simulink subsystem "PvtSubSys_VIE"  (R2020b)
settings: Solver=VariableStepAuto  StartTime=0.0  StopTime=10.0  RelTol=1e-3
undefined symbols (not defined in the file): P_Global_CharSpd_ms, P_Global_FrontAxleToCenter_m, P_Global_RearAxleToCenter_m, P_Global_SideSlipAnglefactor, P_Global_SteeringAngleRatio, P_Global_WheelBase_m, P_Global_WheelTrack_m
libraries: simulink x16
(part 2 of 2)

== matlab function PvtSubSys_VIE/VIE/VIE/VxvRef_Calc/transBrakeToDrive ==
  data: l_tTransBrakeToDrive output; l_tTransDriveToBrake output; axvRefK1 input; axvRef input; vxvRef input; l_tTransBrakeToDriveK1 input single; l_tTransDriveToBrakeK1 input single; l_tHysARefDriveToBrakeInput input single; l_tHysARefBrakeToDriveInput input single; l_tHysARefDriveToBrakeOutput output; l_tHysARefBrakeToDriveOutput output
function [l_tTransBrakeToDrive,l_tTransDriveToBrake,l_tHysARefDriveToBrakeOutput,l_tHysARefBrakeToDriveOutput] = fcn(axvRefK1,axvRef,vxvRef,l_tTransBrakeToDriveK1,l_tTransDriveToBrakeK1,l_tHysARefDriveToBrakeInput,l_tHysARefBrakeToDriveInput)
%#codegen
l_tTransBrakeToDrive = max((l_tTransBrakeToDriveK1-single(0.02)),single(0));  % 常数值转为single型
l_tTransDriveToBrake = max((l_tTransDriveToBrakeK1-single(0.02)),single(0));  % 常数值转为single型

l_tHysARefDriveToBrake=l_tHysARefDriveToBrakeInput;
l_tHysARefBrakeToDrive=l_tHysARefBrakeToDriveInput;

% vsp_checkReinitHys_V
if ((axvRefK1>-0.3)&&(axvRef>-0.3)&&(vxvRef>0))||((axvRefK1<0.3)&&(axvRef<0.3)&&(vxvRef<0)) 
    l_tHysARefDriveToBrake=single(0);% 常数值转为single型
    l_tHysARefBrakeToDrive=single(0);% 常数值转为single型
end
if ((axvRefK1<-0.7)&&(axvRef<-0.7)&&(vxvRef>0))||((axvRefK1>0.7)&&(axvRef>0.7)&&(vxvRef<0)) 
    l_tHysARefDriveToBrake=single(0);% 常数值转为single型
    l_tHysARefBrakeToDrive=single(0);% 常数值转为single型
end   

% vsp_checkStartHys_V
if ((axvRefK1>=-0.3)&&(axvRef<-0.3)&&(vxvRef>0))||((axvRefK1<=0.3)&&(axvRef>0.3)&&(vxvRef<0)) 
   l_tHysARefDriveToBrake = l_tHysARefDriveToBrake + single(0.02);% 常数值转为single型
end
if ((axvRefK1<=-0.7)&&(axvRef>-0.7)&&(vxvRef>0))||((axvRefK1>=0.7)&&(axvRef<0.7)&&(vxvRef<0)) 
   l_tHysARefBrakeToDrive = l_tHysARefBrakeToDrive + single(0.02);% 常数值转为single型
end  

% vsp_checkIncrHys_V
if ((axvRef>=-0.7)&&(axvRef<=-0.3)&&(vxvRef>0))||((axvRef<=0.7)&&(axvRef>=0.3)&&(vxvRef<0)) 
    if l_tHysARefDriveToBrake>0
        l_tHysARefDriveToBrake = min((l_tHysARefDriveToBrake + single(0.02)),single(0.16));% 常数值转为single型
    end
    if l_tHysARefBrakeToDrive>0
        l_tHysARefBrakeToDrive = min((l_tHysARefBrakeToDrive + single(0.02)),single(0.16));% 常数值转为single型
    end
end
%-----------------------------------------------------------------------------------------------%
if ((axvRefK1>=-0.7)&&(axvRef<-0.7)&&(vxvRef>0))||((axvRefK1<=0.7)&&(axvRef>0.7)&&(vxvRef<0))
    if (l_tHysARefDriveToBrake>0)&&(l_tHysARefDriveToBrake<0.16)
        l_tTransDriveToBrake = single(0.15);% 常数值转为single型
    end
end
if ((axvRefK1<=-0.3)&&(axvRef>-0.3)&&(vxvRef>0))||((axvRefK1>=0.3)&&(axvRef<0.3)&&(vxvRef<0))
    if (l_tHysARefBrakeToDrive>0)&&(l_tHysARefBrakeToDrive<0.16)
        l_tTransBrakeToDrive = single(0.15);% 常数值转为single型
    end
end

    l_tHysARefDriveToBrakeOutput=l_tHysARefDriveToBrake;
    l_tHysARefBrakeToDriveOutput=l_tHysARefBrakeToDrive;

== matlab function PvtSubSys_VIE/VIE/VIE/VxvRef_Calc/vsp_calcNoCali_v ==
  data: vxvRef output single; vxwMeanIn input single; l_vxvRefMean input; axvRefLP input single; VehicleStandstill input; axvRefK1 input; axvRef output single
function [vxvRef,axvRef]   = fcn(vxwMeanIn,l_vxvRefMean,axvRefLP,VehicleStandstill,axvRefK1)
%#codegen
vxvRef = l_vxvRefMean;
t_AbsVxwMeanIn = abs(vxwMeanIn);

if t_AbsVxwMeanIn <=0.0039   %%%
    if VehicleStandstill==uint8(1)%转换常数数据类型
        vxvRef=single(0);%转换常数数据类型
        axvRef=single(0);%转换常数数据类型
    else
        axvRef = axvRefK1-single(0.1)*axvRefK1;%转换常数数据类型
    end
else
    axvRef = axvRefLP;
end

== matlab function PvtSubSys_VIE/VIE/VIE/VxvRef_Calc/vsp_filtVxvRefRaw ==
  data: Init input uint8; t_vxvRefRaw input; l_vxvRef input; l_CaseDrive input; l_CaseBrake input; l_tTransDriveToBrake input; l_tTransBrakeToDrive input; vxvRefRaw output; vxvRefRawK1 input single
function vxvRefRaw   = fcn(Init,t_vxvRefRaw,l_vxvRef,l_CaseDrive,l_CaseBrake,l_tTransDriveToBrake,l_tTransBrakeToDrive,vxvRefRawK1)
%#codegen
tFilter=single(1);%转换常数数据类型

if Init==uint8(0)%转换常数数据类型
    if (l_CaseDrive==uint8(0))&&(l_CaseBrake==uint8(0))%转换常数数据类型
        tFilter=single(0.25);%转换常数数据类型
    end
    if (l_tTransDriveToBrake>0)||(l_tTransBrakeToDrive>0)%转换常数数据类型
        tFilter=single(0.125);%转换常数数据类型
    end

    vxvRefRaw = vxvRefRawK1 + tFilter*(t_vxvRefRaw - vxvRefRawK1);

    t_temp1 = abs(vxvRefRaw);
    t_temp2 = abs(l_vxvRef);

    if ((l_CaseBrake==uint8(1))&&(t_temp1>t_temp2))||((l_CaseDrive==uint8(1))&&(t_temp1<t_temp2))%转换常数数据类型
       vxvRefRaw = l_vxvRef;
    end


    t_temp1 = single(0.24);%转换常数数据类型
    t_temp2 = vxvRefRawK1 + t_temp1;
    t_temp3 = vxvRefRawK1 - t_temp1;

    t_temp1 = min(vxvRefRaw,t_temp2);
    vxvRefRaw = max(t_temp1,t_temp3);
else
    vxvRefRaw = t_vxvRefRaw;
end

== matlab function PvtSubSys_VIE/VIE/VIE/alpSumSlideCurveness ==
  data: vRef input; alpSumSlideCurveness output; psiDtOpt input; alpSumSlideCurvenessK1 input single
function alpSumSlideCurveness = fcn(vRef,psiDtOpt,alpSumSlideCurvenessK1)

if abs(vRef)<0.01
   t_tauCurveness = single(65535);%转换常数数据类型
else
   t_tauCurveness = min(400/abs(vRef),single(65535));%转换常数数据类型
end
% t_tauKapDtCurvenessUp = t_tauCurveness/8;
% t_tauKapDtCurvenessDown = t_tauCurveness/2;

temp1 = single(abs(psiDtOpt));%abs(psiDtOpt)转为single型
if temp1<0.003
   temp1 = single(0); %转换常数数据类型
end
temp2 = alpSumSlideCurvenessK1/t_tauCurveness;
temp2 = temp1 - temp2;
temp3 = single(0.02)*temp2;%转换常数数据类型
alpSumSlideCurveness = min(alpSumSlideCurvenessK1 + temp3,single(2));%转换常数数据类型

end

== matlab function PvtSubSys_VIE/VIE/VIE/VxvRef_Calc/VxvRef_Calc/MATLAB Function2 ==
  data: y output; SteerAngleOffset_deg input single; SteerAngOffsetInit input single
function y  = fcn(SteerAngleOffset_deg,SteerAngOffsetInit)

persistent T
if isempty(T)
    T = single(0);
end

t = single(0.02);
T = min(T+t,1000);
if T > 0.1
    y = SteerAngleOffset_deg;       
else
    y = SteerAngOffsetInit;
end

end

== matlab function PvtSubSys_VIE/VIE/VIE/AxRef/MATLAB Function ==
  data: AxvS input; Ax output; AxvRef input; VxvRef input; Error input; AxK1 input single
function Ax = fcn(AxvS,AxvRef,VxvRef,Error,AxK1)
%#codegen
if (AxvRef==uint8(0))&&(VxvRef==uint8(0))%转换常数数据类型
    Ax=single(0);%转换常数数据类型
else
   if abs(AxvS-AxvRef)<Error
       AxRaw = single(0.5)*(AxvS+AxvRef);%转换常数数据类型
   else
       AxRaw = AxvRef;
   end
    Ax = single(0.25)*(AxRaw-AxK1) + AxK1;%转换常数数据类型
end

== matlab function PvtSubSys_VIE/VIE/VIE/PsiDtStandstillCalc/MATLAB Function ==
  data: AlpDtSteerAngle input single; PsiDtLP output single; PsiDtInF input single; Standstill input boolean; PsiDtDt input; PsiDtDtLP input single; PsiDtLPK1 input; PsiDtStandstillK1 input; PsiDtStandstill output single
function [PsiDtLP,PsiDtStandstill] = PsiDtStandstillCalc(AlpDtSteerAngle,PsiDtInF,Standstill,PsiDtDt,PsiDtDtLP,PsiDtLPK1,PsiDtStandstillK1)
%#codegen
PsiDtStandstill = PsiDtStandstillK1;
PsiDtLP = PsiDtLPK1;
tauLPStill = single(0.02)/single(0.5);%转换常数数据类型
tauLPStandStill = single(0.02)/single(5);%转换常数数据类型
PsiDtLP = PsiDtLP + tauLPStill*(PsiDtInF-PsiDtLP);
if (Standstill==1)&&...
        (abs(PsiDtLP)<0.08)&&...
        (abs(PsiDtDt)<0.1)&&...
        (abs(PsiDtDtLP)<0.01)&&...
        (abs(AlpDtSteerAngle)<=1.5708)
    PsiDtStandstill = PsiDtStandstill + tauLPStandStill*(PsiDtInF-PsiDtStandstill);
end

== matlab function PvtSubSys_VIE/VIE/VIE/VxvRef_Calc/VxvRef_Calc/YOD_Ackman ==
  data: AckConst output; VxvRef input; Vch input; WheelBase input; AlpWheelAngle input; PsiDtAckK1 input single; PsiDtAck output
function [AckConst,PsiDtAck] = Ackman(VxvRef,Vch,WheelBase,AlpWheelAngle,PsiDtAckK1)
%#codegen
if VxvRef==uint8(0)%转换常数数据类型
    PsiDtAckRaw = single(0);%转换常数数据类型
    AckConst = single(1);%转换常数数据类型
else
    AckConst = min((single(1)+VxvRef*VxvRef/(Vch*Vch))*WheelBase/VxvRef,single(32767));%转换常数数据类型
    PsiDtAckRaw = AlpWheelAngle/AckConst;
end
PsiDtAck = (single(0.02/0.1))*(PsiDtAckRaw-PsiDtAckK1)+PsiDtAckK1;%转换常数数据类型

== matlab function PvtSubSys_VIE/VIE/VIE/VxvRef_Calc/VxwCorr ==
  data: VxwFL input single; vxwCorrFL output; VxwFR input single; VxwRL input single; VxwRR input single; L1 input; L2 input; Yawrate input; alpAngle input; b input; vxwCorrFR output; vxwCorrRL output; vxwCorrRR output
function [vxwCorrFL,vxwCorrFR,vxwCorrRL,vxwCorrRR] = fcn(VxwFL,VxwFR,VxwRL,VxwRR,L1,L2,Yawrate,alpAngle,b)
%#codegen

vxwCorrFL = (VxwFL-(L1+L2)*Yawrate*sin(alpAngle))/cos(alpAngle) + b*Yawrate/single(2); %常数转为single类型

vxwCorrFR = (VxwFR-(L1+L2)*Yawrate*sin(alpAngle))/cos(alpAngle) - b*Yawrate/single(2);%常数转为single类型

vxwCorrRL = VxwRL + b*Yawrate/single(2);%常数转为single类型

vxwCorrRR = VxwRR - b*Yawrate/single(2);%常数转为single类型

== matlab function PvtSubSys_VIE/VIE/VIE/VxvRef_Calc/calcBrakeDriveState ==
  data: axvTrend input; l_CaseDrive output uint8; axvRef input; vxvRef input; l_CaseBrake output uint8; t_SlipDrive output single; t_SlipBrake output single; l_tTransDriveToBrake input
function [l_CaseDrive,l_CaseBrake,t_SlipDrive,t_SlipBrake] = fcn(axvTrend,axvRef,vxvRef,l_tTransDriveToBrake)
%#codegen

   if ( (axvTrend > 0.5)&&(axvRef> 0.5) &&(vxvRef> 0 )) || ((axvTrend< -0.5) &&(axvRef< -0.5) &&(vxvRef  < 0 ))
      l_CaseDrive = uint8(1); %l_CaseDrive赋的常数值转为uint8型
   else
      l_CaseDrive = uint8(0);%l_CaseDrive赋的常数值转为uint8型
   end
   
   if ( (axvTrend < -0.5)&&(axvRef< -0.5) &&(vxvRef> 0 )) || ((axvTrend> 0.5) &&(axvRef> 0.5) &&(vxvRef  < 0 ))
      l_CaseBrake = uint8(1);%l_CaseBrake赋的常数值转为uint8型
   else
      l_CaseBrake = uint8(0);%l_CaseBrake赋的常数值转为uint8型
   end
   
   t=abs(axvRef);
   
   if t>=0.5
       t=t-single(0.5); %常数转为single型
       t_Slip = single(0.00815)*t;%常数转为single型
   else
       t_Slip=single(0);%常数转为single型
   end
   
   if l_CaseDrive==uint8(1)    %常数值转为uint8型
       t_SlipDrive = -t_Slip;
       t_SlipBrake = single(0); %常数值转为single型
   else
      t_SlipDrive=single(0); %常数值转为single型
      if (l_CaseBrake==uint8(1))&&(l_tTransDriveToBrake==uint8(0))  %常数值转为uint8型
          t_SlipBrake = t_Slip;
      else
          t_SlipBrake =single(0);%常数值转为single型
      end       
   end
